simulink library "NeuroMuscularLibrary2"  (R2019b)
settings: Solver=ode45  StartTime=0.0  StopTime=10.0  RelTol=1e-3  EnableMultiTasking=on
values from neighbouring files (symbols this model uses):
  c = 0.05    [BodyMechParams.m]
  c_jointstop = 0.3 / (pi/180)    (= 17.1887338539)    [BodyMechParams.m]
  deltaLegAngleThr = 8*pi/180    (= 0.13962634016)    [CMGParams.m]
  DeltaThRef = 2e-3    (= 0.002)    [BodyMechParams.m]
  eref = 0.04    [BodyMechParams.m]
  FmaxGLU = 1500    [BodyMechParams.m]
  footBallToAnkleDist = 0.16    [BodyMechParams.m]
  footBallToCenterDist = footLength/2    (= 0.1)    [BodyMechParams.m]
  footBallToHeelDist = footLength    (= 0.2)    [BodyMechParams.m]
  footCenterToCGDist = 0.14 - footBallToCenterDist    (= 0.04)    [BodyMechParams.m]
  footInertia = 0.005    [BodyMechParams.m]
  footLength = 0.2    [BodyMechParams.m]
  footMass = 1.25    [BodyMechParams.m]
  FT_GLU = 47.6    [BodyMechParams.m]
  g = 9.80665    [BodyMechParams.m]
  groundTheta = [atan(diff(groundZ)./diff(groundX)), 0]    [generateGround.m]
  groundZ = groundZ * stepSize/(largestStep+eps)    [generateGround.m]
  hatHipToCenterDistLen = hatLength/2    (= 0.4)    [BodyMechParams.m]
  hatInertia = 3    [BodyMechParams.m]
  hatLeftHipToCenterDistWidth = .15    (= 0.15)    [BodyMechParams.m]
  hatLength = 0.8    [BodyMechParams.m]
  hatMass = 53.5    [BodyMechParams.m]
  hatThickness = 0.2    [BodyMechParams.m]
  hatWidth = 0.4    [BodyMechParams.m]
  K = 5    [BodyMechParams.m]
  k_gn = k_gn/2    (= 39226.6)    [BodyMechParams.m]
  k_gt = k_gt/2    (= 39226.6)    [BodyMechParams.m]
  k_pressure = hatMass * g / DeltaThRef    (= 262327.8875)    [BodyMechParams.m]
  legAngleSpeedMax = 10    [CMGParams.m]
  loptGAS = 0.05    [BodyMechParams.m]
  loptGLU = 0.11    [BodyMechParams.m]
  loptHAB = 0.09    [BodyMechParams.m]
  loptHAD = 0.10    (= 0.1)    [BodyMechParams.m]
  loptHAM = 0.10    (= 0.1)    [BodyMechParams.m]
  loptHFL = 0.11    [BodyMechParams.m]
  loptSOL = 0.04    [BodyMechParams.m]
  loptTA = 0.06    [BodyMechParams.m]
  loptVAS = 0.08    [BodyMechParams.m]
  lslackGAS = 0.40    (= 0.4)    [BodyMechParams.m]
  lslackGLU = 0.13    [BodyMechParams.m]
  lslackHAB = 0.07    [BodyMechParams.m]
  lslackHAD = 0.18    [BodyMechParams.m]
  lslackHAM = 0.31    [BodyMechParams.m]
  lslackHFL = 0.10    (= 0.1)    [BodyMechParams.m]
  lslackSOL = 0.26    [BodyMechParams.m]
  lslackTA = 0.24    [BodyMechParams.m]
  lslackVAS = 0.23    [BodyMechParams.m]
  mu_slide = 0.8    [BodyMechParams.m]
  mu_stick = 0.9    [BodyMechParams.m]
  N = 1.5    [BodyMechParams.m]    (also in cmaes.m = size(x,1); mergeCompareEnergyCosts.m = {S.name})
  phiKneeUpLimit = 5*pi/180    (= 0.0872664625997)    [BodyMechParams.m]
  phimaxGASa = 20*pi/180    (= 0.349065850399)    [BodyMechParams.m]
  phimaxGASk = 40*pi/180    (= 0.698131700798)    [BodyMechParams.m]
  phimaxHAMk = 0*pi/180    (= 0)    [BodyMechParams.m]
  phimaxSOL = 20*pi/180    (= 0.349065850399)    [BodyMechParams.m]
  phimaxTA = -10*pi/180    (= -0.174532925199)    [BodyMechParams.m]
  phimaxVAS = 15*pi/180    (= 0.261799387799)    [BodyMechParams.m]
  phirefGASa = -10*pi/180    (= -0.174532925199)    [BodyMechParams.m]
  phirefGASk = 15*pi/180    (= 0.261799387799)    [BodyMechParams.m]
  phirefGLU = -30*pi/180    (= -0.523598775598)    [BodyMechParams.m]
  phirefHAB = 10*pi/180    (= 0.174532925199)    [BodyMechParams.m]
  phirefHAD = 15*pi/180    (= 0.261799387799)    [BodyMechParams.m]
  phirefHAMh = -25*pi/180    (= -0.436332312999)    [BodyMechParams.m]
  phirefHAMk = 0*pi/180    (= 0)    [BodyMechParams.m]
  phirefHFL = 0*pi/180    (= 0)    [BodyMechParams.m]
  phirefSOL = -10*pi/180    (= -0.174532925199)    [BodyMechParams.m]
  phirefTA = 20*pi/180    (= 0.349065850399)    [BodyMechParams.m]
  phirefVAS = 55*pi/180    (= 0.959931088597)    [BodyMechParams.m]
  rGASa = 0.05    [BodyMechParams.m]
  rGASk = 0.05    [BodyMechParams.m]
  rGLU = 0.10    (= 0.1)    [BodyMechParams.m]
  rHAB = 0.06    [BodyMechParams.m]
  rHAD = 0.03    [BodyMechParams.m]
  rHAMh = 0.08    [BodyMechParams.m]
  rHAMk = 0.05    [BodyMechParams.m]
  rHFL = 0.10    (= 0.1)    [BodyMechParams.m]
  rhoGASa = 0.7    [BodyMechParams.m]
  rhoGASk = 0.7    [BodyMechParams.m]
  rhoGLU = 0.5    [BodyMechParams.m]
  rhoHAB = 0.7    [BodyMechParams.m]
  rhoHAD = 1    [BodyMechParams.m]
  rhoHAMh = 0.7    [BodyMechParams.m]
  rhoHAMk = 0.7    [BodyMechParams.m]
  rhoHFL = 0.5    [BodyMechParams.m]
  rhoSOL = 0.5    [BodyMechParams.m]
  rhoTA = 0.7    [BodyMechParams.m]
  rhoVAS = 0.7    [BodyMechParams.m]
  RkneeExtendGain = 25000    [CMGParams.m]
  RkneeStopGain = 12000    [CMGParams.m]
  RlegAngleFilter = 100    [CMGParams.m]
  rSOL = 0.05    [BodyMechParams.m]
  rTA = 0.04    [BodyMechParams.m]
  rVAS = 0.06    [BodyMechParams.m]
  s = x(1:N-1,:).^2 + x(2:N,:).^2    [cmaes.m]
  shankAnkleToCenterDist = shankLength/2    (= 0.25)    [BodyMechParams.m]
  shankAnkleToKneeDist = shankLength    (= 0.5)    [BodyMechParams.m]
  shankCenterToCGDist = 0.3 - shankAnkleToCenterDist    (= 0.05)    [BodyMechParams.m]
  shankInertia = 0.05    [BodyMechParams.m]
  shankLength = 0.5    [BodyMechParams.m]
  shankMass = 3.5    [BodyMechParams.m]
  tau = 0.01    [BodyMechParams.m]
  thighCenterToCGDist = 0.3 - thighKneeToCenterDist    (= 0.05)    [BodyMechParams.m]
  thighInertia = 0.15    [BodyMechParams.m]
  thighKneeToCenterDist = thighLength/2    (= 0.25)    [BodyMechParams.m]
  thighKneeToHipDist = thighLength    (= 0.5)    [BodyMechParams.m]
  thighLength = 0.5    [BodyMechParams.m]
  thighMass = 8.5    [BodyMechParams.m]
  v_gn_max = v_gz_max    (= 0.03)    [BodyMechParams.m]
  v_gt_max = v_gz_max    (= 0.03)    [BodyMechParams.m]
  v_max_pressure = 0.5    [BodyMechParams.m]
  vLimit = 0.01    [BodyMechParams.m]
  w = 0.56    [BodyMechParams.m]    (also in MuscleEnergyTest.m = 1.039; cmaes.m = ones(size(x,1)))
  w_max_jointstop = 1 * pi/180    (= 0.0174532925199)    [BodyMechParams.m]
  X = contains(N,'compareEnergyCost') .* ~contains(N,'total') .* ~contains(N,'Total')    [mergeCompareEnergyCosts.m]
undefined symbols (not defined in the file or in its folder): abdHATRef, ankleBackDriveGain, ankleCJointstop, ankleDgain, ankleFilterPID, ankleFilterSEA, ankleGearEff, ankleGearRatio, ankleIgain, ankleInitialAngle, ankleInputMass, ankleIntCoulomb, ankleIntDamping, ankleIntStatic, ankleParallelSpringDamping, ankleParallelSpringOffset, ankleParallelSpringStiffness, anklePgain, anklePlantarLimit, ankleSEADamping, ankleSEAStiffness, ankleTendonMass, ankleWMaxJointstop, dryFrictionDamping, dryFrictionStiffness, dryFrictionVelThresh, footMassp, FourBarL1, FourBarL3, GainCHAB, GainCHAD, GainGAS, GainGLU, GainHAM, GainKneeOverExt, GainSOL, GainSOLTA, GainTA, GainVAS, hipDGain, hipDGainAbd, hipPGain, hipPGainAbd, Kglu, kneeAngleOffset, kneeBackDriveGain, kneeCJointstop, kneeDgain, kneeExtCoulomb, kneeExtDamping, kneeExtendGain, kneeExtStatic, kneeFilterPID, kneeFilterSEA, kneeFlexGain, kneeGearEff, kneeGearRatio, kneeHoldGain1, kneeHoldGain2, kneeIgain ... (+62)
libraries: sm_lib x105, nesl_utility x55, simulink x22, dspswit3 x15, $bdroot x12, simulink_extras x2
(part 3 of 6)

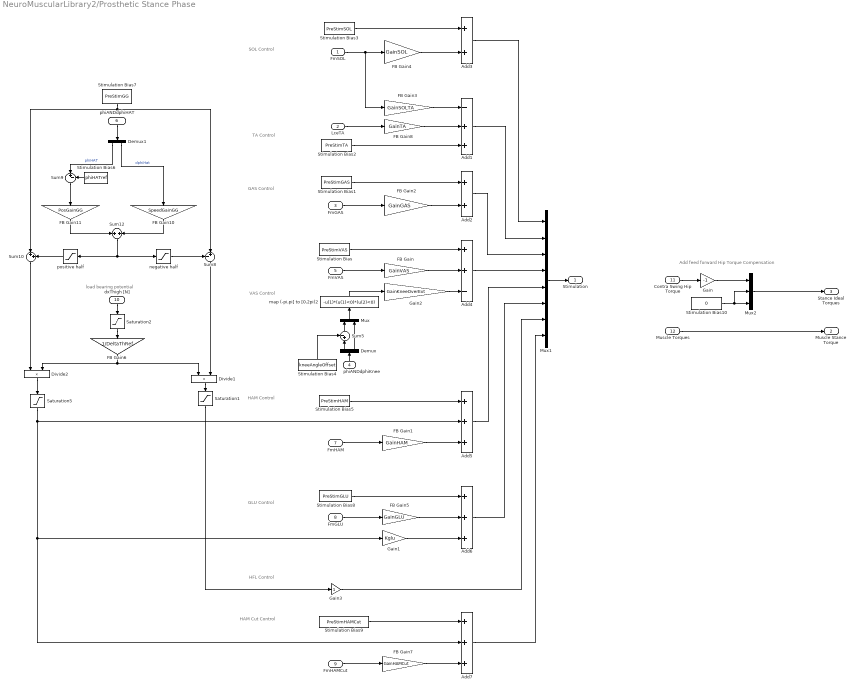
== system NeuroMuscularLibrary2/Prosthetic Stance Phase ==
  note: Add feed forward Hip Torque Compensation
  note: load bearing potential
  note: HFL Control
  note: GLU Control
  note: VAS Control
  note: HAM Control
  note: GAS Control
  note: TA Control
  note: SOL Control
  note: HAM Cut Control
  FmSOL : Inport
  LceTA : Inport  Port=2
  FmGAS : Inport  Port=3
  phiANDdphiKnee : Inport  Port=4
  FmVAS : Inport  Port=5
  phiANDdphiHAT : Inport  Port=6
  FmHAM : Inport  Port=7
  FmGLU : Inport  Port=8
  FmHAMCut : Inport  Port=9
  dxThigh [N] : Inport  Port=10
  Contra Swing Hip Torque : Inport  Port=11
  Muscle Torques : Inport  Port=12
  Add1 : Sum  Inputs=-++
  Add2 : Sum
  Add3 : Sum
  Add4 : Sum  Inputs=++-
  Add5 : Sum  Inputs=+++
  Add6 : Sum  Inputs=+++
  Add7 : Sum  Inputs=+++
  Demux : Demux  Outputs=2
  Demux1 : Demux  Outputs=2
  Divide1 : Product
  Divide2 : Product
  FB Gain : Gain  Gain=GainVAS  SaturateOnIntegerOverflow=on  OutDataTypeStr=Inherit: Same as input  ParamDataTypeStr=Inherit: Same as input
  FB Gain1 : Gain  Gain=GainHAM  SaturateOnIntegerOverflow=on  OutDataTypeStr=Inherit: Same as input  ParamDataTypeStr=Inherit: Same as input
  FB Gain10 : Gain  Gain=SpeedGainGG  SaturateOnIntegerOverflow=on  OutDataTypeStr=Inherit: Same as input  ParamDataTypeStr=Inherit: Same as input
  FB Gain11 : Gain  Gain=PosGainGG  SaturateOnIntegerOverflow=on  OutDataTypeStr=Inherit: Same as input  ParamDataTypeStr=Inherit: Same as input
  FB Gain2 : Gain  Gain=GainGAS  SaturateOnIntegerOverflow=on  OutDataTypeStr=Inherit: Same as input  ParamDataTypeStr=Inherit: Same as input
  FB Gain3 : Gain  Gain=GainSOLTA  SaturateOnIntegerOverflow=on  OutDataTypeStr=Inherit: Same as input  ParamDataTypeStr=Inherit: Same as input
  FB Gain4 : Gain  Gain=GainSOL  SaturateOnIntegerOverflow=on  OutDataTypeStr=Inherit: Same as input  ParamDataTypeStr=Inherit: Same as input
  FB Gain5 : Gain  Gain=GainGLU  SaturateOnIntegerOverflow=on  OutDataTypeStr=Inherit: Same as input  ParamDataTypeStr=Inherit: Same as input
  FB Gain6 : Gain  Gain=1/DeltaThRef  SaturateOnIntegerOverflow=on  OutDataTypeStr=Inherit: Same as input  ParamDataTypeStr=Inherit: Same as input
  FB Gain7 : Gain  Gain=GainHAMCut  SaturateOnIntegerOverflow=on  OutDataTypeStr=Inherit: Same as input  ParamDataTypeStr=Inherit: Same as input
  FB Gain8 : Gain  Gain=GainTA  SaturateOnIntegerOverflow=on  OutDataTypeStr=Inherit: Same as input  ParamDataTypeStr=Inherit: Same as input
  Gain : Gain  Gain=-1
  Gain1 : Gain  Gain=Kglu
  Gain2 : Gain  Gain=GainKneeOverExt
  Gain3 : Gain
  Mux : Mux  Inputs=2
  Mux1 : Mux  Inputs=8
  Mux2 : Mux  Inputs=3
  Saturation1 : Saturate  UpperLimit=1  LowerLimit=0  ZeroCross=off
  Saturation2 : Saturate  UpperLimit=inf  LowerLimit=0  ZeroCross=off
  Saturation5 : Saturate  UpperLimit=1  LowerLimit=0  ZeroCross=off
  Stimulation Bias : Constant  Value=PreStimVAS
  Stimulation Bias1 : Constant  Value=PreStimGAS
  Stimulation Bias10 : Constant  Value=0
  Stimulation Bias2 : Constant  Value=PreStimTA
  Stimulation Bias3 : Constant  Value=PreStimSOL
  Stimulation Bias4 : Constant  Value=kneeAngleOffset
  Stimulation Bias5 : Constant  Value=PreStimHAM
  Stimulation Bias6 : Constant  Value=phiHATref
  Stimulation Bias7 : Constant  Value=PreStimGG
  Stimulation Bias8 : Constant  Value=PreStimGLU
  Stimulation Bias9 : Constant  Value=PreStimHAMCut
  Sum10 : Sum  Inputs=|++  SaturateOnIntegerOverflow=on  InputSameDT=on  OutDataTypeStr=Inherit: Same as first input
  Sum12 : Sum  SaturateOnIntegerOverflow=on  InputSameDT=on  OutDataTypeStr=Inherit: Same as first input
  Sum5 : Sum  Inputs=-+|  SaturateOnIntegerOverflow=on  InputSameDT=on  OutDataTypeStr=Inherit: Same as first input
  Sum8 : Sum  Inputs=-+|  SaturateOnIntegerOverflow=on  InputSameDT=on  OutDataTypeStr=Inherit: Same as first input
  Sum9 : Sum  Inputs=|+-  SaturateOnIntegerOverflow=on  InputSameDT=on  OutDataTypeStr=Inherit: Same as first input
  map (-pi,pi] to [0,2pi)2 : Fcn  Expr=-u(1)*(u(1)<0)*(u(2)<0)
  negative half : Saturate  UpperLimit=0  LowerLimit=-inf  ZeroCross=off
  positive half : Saturate  UpperLimit=inf  LowerLimit=0  ZeroCross=off
  Stimulation : Outport
  Muscle Stance Torque : Outport  Port=2
  Stance Ideal Torques : Outport  Port=3
  wires:
  Muscle Torques/1 -> Muscle Stance Torque/1
  Mux2/1 -> Stance Ideal Torques/1
  Stimulation Bias10/1 -> Mux2/2, Mux2/3
  Contra Swing Hip Torque/1 -> Gain/1
  Gain/1 -> Mux2/1
  Add4/1 -> Mux1/4
  Mux1/1 -> Stimulation/1
  Gain1/1 -> Add6/3
  FB Gain5/1 -> Add6/2
  Stimulation Bias8/1 -> Add6/1
  Add6/1 -> Mux1/6
  Add5/1 -> Mux1/5
  FB Gain1/1 -> Add5/3
  Stimulation Bias5/1 -> Add5/1
  Stimulation Bias/1 -> Add4/1
  Stimulation Bias1/1 -> Add2/1
  Add2/1 -> Mux1/3
  Stimulation Bias2/1 -> Add1/3
  Stimulation Bias3/1 -> Add3/1
  FmGLU/1 -> FB Gain5/1
  FmHAM/1 -> FB Gain1/1
  map (-pi,pi] to [0,2pi)2/1 -> Gain2/1
  Sum8/1 -> Divide1/2
  Sum10/1 -> Divide2/1
  Sum9/1 -> FB Gain11/1
  FB Gain6/1 -> Divide1/1, Divide2/2
  Divide2/1 -> Saturation5/1
  Divide1/1 -> Saturation1/1
  Saturation1/1 -> Gain3/1
  dxThigh [N]/1 -> Saturation2/1
  Saturation2/1 -> FB Gain6/1
  Gain3/1 -> Mux1/7
  Gain2/1 -> Add4/3
  negative half/1 -> Sum8/1
  Sum12/1 -> negative half/1, positive half/1
  positive half/1 -> Sum10/2
  Demux1/2 -> FB Gain10/1  "dphiHat"
  Demux1/1 -> Sum9/1  "phiHAT"
  phiANDdphiHAT/1 -> Demux1/1
  FB Gain10/1 -> Sum12/2
  FB Gain11/1 -> Sum12/1
  Stimulation Bias7/1 -> Sum8/2, Sum10/1
  Stimulation Bias6/1 -> Sum9/2
  Stimulation Bias4/1 -> Sum5/1
  Demux/2 -> Mux/2
  Demux/1 -> Sum5/2
  phiANDdphiKnee/1 -> Demux/1
  Sum5/1 -> Mux/1
  Mux/1 -> map (-pi,pi] to [0,2pi)2/1
  FmVAS/1 -> FB Gain/1
  FB Gain/1 -> Add4/2
  FB Gain2/1 -> Add2/2
  FmGAS/1 -> FB Gain2/1
  LceTA/1 -> FB Gain8/1
  FB Gain8/1 -> Add1/2
  Add1/1 -> Mux1/2
  FB Gain3/1 -> Add1/1
  FmSOL/1 -> FB Gain3/1, FB Gain4/1
  FB Gain4/1 -> Add3/2
  Add3/1 -> Mux1/1
  Add7/1 -> Mux1/8
  FB Gain7/1 -> Add7/3
  Stimulation Bias9/1 -> Add7/1
  FmHAMCut/1 -> FB Gain7/1
  Saturation5/1 -> Add5/2, Add7/2, Gain1/1

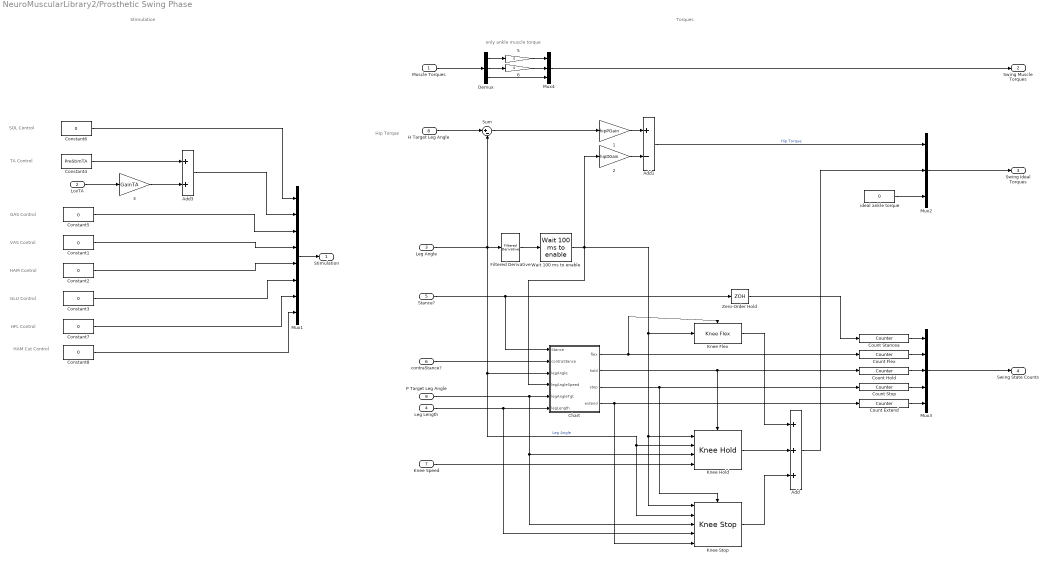
== system NeuroMuscularLibrary2/Prosthetic Swing Phase ==
  note: Hip Torque
  note: only ankle muscle torque
  note: HAM Cut
      | Control
  note: Torques
  note: HFL Control
  note: GLU Control
  note: HAM Control
  note: VAS Control
  note: TA Control
  note: GAS Control
  note: SOL Control
  note: Stimulation
  Muscle Torques : Inport
  LceTA : Inport  Port=2
  Leg Angle : Inport  Port=3
  Leg Length : Inport  Port=4
  Stance? : Inport  Port=5
  contraStance? : Inport  Port=6
  Knee Speed : Inport  Port=7
  H Target Leg Angle : Inport  Port=8
  P Target Leg Angle : Inport  Port=9
  " 1" : Gain  Gain=hipPGain
  " 2" : Gain  Gain=hipDGain
  " 3" : Gain  Gain=GainTA
  " 5" : Gain  Gain=0
  " 6" : Gain  Gain=0
  Add : Sum  Inputs=+++
  Add1 : Sum  Inputs=+-
  Add3 : Sum
  Chart : Stateflow chart  TreatAsAtomicUnit=on
  Constant{1..3,5..8} (7 alike) : Constant  Value=0
  Constant4 : Constant  Value=PreStimTA
  Count Extend : dspswit3/Counter  Direction=Up  CountEvent=Rising edge  CounterSize=16 bits  MaxCount=255  InitialCount=0  Output=Count  HitValue=32  ResetInput=off  SamplesPerFrame=1  Ts=1  CntDtype=double  HitDtype=Logical
  Count Flex : dspswit3/Counter  Direction=Up  CountEvent=Rising edge  CounterSize=16 bits  MaxCount=255  InitialCount=0  Output=Count  HitValue=32  ResetInput=off  SamplesPerFrame=1  Ts=1  CntDtype=double  HitDtype=Logical
  Count Hold : dspswit3/Counter  Direction=Up  CountEvent=Rising edge  CounterSize=16 bits  MaxCount=255  InitialCount=0  Output=Count  HitValue=32  ResetInput=off  SamplesPerFrame=1  Ts=1  CntDtype=double  HitDtype=Logical
  Count Stancea : dspswit3/Counter  Direction=Up  CountEvent=Rising edge  CounterSize=16 bits  MaxCount=255  InitialCount=0  Output=Count  HitValue=32  ResetInput=off  SamplesPerFrame=1  Ts=1  CntDtype=double  HitDtype=Logical
  Count Stop : dspswit3/Counter  Direction=Up  CountEvent=Rising edge  CounterSize=16 bits  MaxCount=255  InitialCount=0  Output=Count  HitValue=32  ResetInput=off  SamplesPerFrame=1  Ts=1  CntDtype=double  HitDtype=Logical
  Demux : Demux  Outputs=3
  Filtered Derivative : $bdroot/Swing Phase/Filtered Derivative  SystemSampleTime=-1  Latency=0  AutoFrameSizeCalculation=off
  Knee Flex : $bdroot/Swing Phase/Knee Flex  SystemSampleTime=-1  Latency=0  AutoFrameSizeCalculation=off
  Knee Hold : $bdroot/Swing Phase/Knee Hold  SystemSampleTime=-1  Latency=0  AutoFrameSizeCalculation=off
  Knee Stop : $bdroot/Swing Phase/Knee Stop  SystemSampleTime=-1  Latency=0  AutoFrameSizeCalculation=off
  Mux1 : Mux  Inputs=8
  Mux2 : Mux  Inputs=3
  Mux3 : Mux  Inputs=5
  Mux4 : Mux  Inputs=3
  Sum : Sum  Inputs=|+-
  Wait 100 ms to enable : $bdroot/Swing Phase/Wait 100 ms to enable  SystemSampleTime=-1  Latency=0  AutoFrameSizeCalculation=off
  Zero-Order Hold : ZeroOrderHold  SampleTime=.01
  ideal ankle torque : Constant  Value=0
  Stimulation : Outport
  Swing Muscle Torques : Outport  Port=2
  Swing Ideal Torques : Outport  Port=3
  Swing State Counts : Outport  Port=4
  wires:
  P Target Leg Angle/1 -> Chart/5(legAngleTgt), Knee Hold/3, Knee Stop/3
  Mux2/1 -> Swing Ideal Torques/1
  ideal ankle torque/1 -> Mux2/3
  Zero-Order Hold/1 -> Count Stancea/1
  Count Stancea/1 -> Mux3/1
  Mux3/1 -> Swing State Counts/1
  Count Flex/1 -> Mux3/2
  Count Hold/1 -> Mux3/3
  Count Stop/1 -> Mux3/4
  Count Extend/1 -> Mux3/5
  Add1/1 -> Mux2/1  "Hip Torque"
  Leg Length/1 -> Knee Stop/4, Chart/6(legLength)
  contraStance?/1 -> Chart/2(contraStance)
  Stance?/1 -> Chart/1(Stance), Zero-Order Hold/1
  Chart/4(extend) -> Knee Stop/5, Count Extend/1
  Chart/3(stop) -> Knee Stop/Enable, Count Stop/1
  Chart/2(hold) -> Knee Hold/Enable, Count Hold/1
  Chart/1(flex) -> Count Flex/1, Knee Flex/Enable
  Add/1 -> Mux2/2
  Knee Stop/1 -> Add/3
  Knee Flex/1 -> Add/1
  Knee Hold/1 -> Add/2
  Knee Speed/1 -> Knee Hold/4
  Leg Angle/1 -> Sum/2, Knee Hold/2, Knee Stop/2, Chart/3(legAngle), Filtered Derivative/1  "Leg Angle"
  Sum/1 -> " 1"/1
  " 1"/1 -> Add1/1
  " 2"/1 -> Add1/2
  H Target Leg Angle/1 -> Sum/1
  Filtered Derivative/1 -> Wait 100 ms to enable/1
  Wait 100 ms to enable/1 -> " 2"/1, Knee Flex/1, Knee Stop/1, Knee Hold/1, Chart/4(legAngleSpeed)
  Demux/3 -> Mux4/3
  " 6"/1 -> Mux4/2
  " 5"/1 -> Mux4/1
  Demux/2 -> " 6"/1
  Demux/1 -> " 5"/1
  Muscle Torques/1 -> Demux/1
  Mux4/1 -> Swing Muscle Torques/1
  Constant8/1 -> Mux1/8
  Mux1/1 -> Stimulation/1
  Constant7/1 -> Mux1/7
  Constant3/1 -> Mux1/6
  Constant2/1 -> Mux1/5
  Constant1/1 -> Mux1/4
  Constant5/1 -> Mux1/3
  Constant6/1 -> Mux1/1
  Add3/1 -> Mux1/2
  LceTA/1 -> " 3"/1
  " 3"/1 -> Add3/2
  Constant4/1 -> Add3/1

== system NeuroMuscularLibrary2/SOL Link ==
  note: Soleus Attachment
  Ankle Angle [rad] : Inport
  Constant : Constant  Value=lslackSOL+loptSOL
  Constant2 : Constant  Value=phirefSOL
  Constant3 : Constant  Value=phimaxSOL
  Demux : Demux  Outputs=2
  Gain2 : Gain  Gain=rSOL
  Gain4 : Gain  Gain=rhoSOL
  Mux : Mux  Inputs=2
  Sum2 : Sum  Inputs=|+-
  Sum3 : Sum  Inputs=-+|
  Sum4 : Sum  Inputs=+-
  Sum5 : Sum  Inputs=|++
  length change term : Trigonometry
  offset correction term : Trigonometry
  variable lever term : Trigonometry  Operator=cos
  lmtc [m] : Outport
  lever [m] : Outport  Port=2
  wires:
  Ankle Angle [rad]/1 -> Sum3/2
  Sum3/1 -> variable lever term/1, length change term/1
  Constant3/1 -> Sum3/1, Sum2/2
  Sum2/1 -> offset correction term/1
  Constant2/1 -> Sum2/1
  length change term/1 -> Sum4/2
  offset correction term/1 -> Sum4/1
  Sum4/1 -> Mux/1
  Constant/1 -> Sum5/1
  Sum5/1 -> lmtc [m]/1
  Gain4/1 -> Sum5/2
  variable lever term/1 -> Mux/2
  Mux/1 -> Gain2/1
  Gain2/1 -> Demux/1
  Demux/1 -> Gain4/1
  Demux/2 -> lever [m]/1

== system NeuroMuscularLibrary2/Sensor Sheet ==
  note: Inner Segment Pressure Sheet
  Gain3 : Gain  Gain=k_pressure
  Gain4 : Gain  Gain=1/v_max_pressure
  Mux1 : Mux  Inputs=2
  PS-Simulink Converter : nesl_utility/PS-Simulink Converter  PhysicalDomain=network_engine_domain  SubClassName=ps_output  LeftPortType=input  RightPortType=output  PseudoPeriodic=off  Frequencies=[]  Unit=1  AffineConversion=off
  PS-Simulink Converter1 : nesl_utility/PS-Simulink Converter  PhysicalDomain=network_engine_domain  SubClassName=ps_output  LeftPortType=input  RightPortType=output  PseudoPeriodic=off  Frequencies=[]  Unit=1  AffineConversion=off
  Pressure Sheet Reaction Force : Fcn  Expr=-u(1) * (1+sgn(u(1))*u(2))
  Prismatic Joint : sm_lib/Joints/Prismatic Joint  JointMode=Normal  SenseConstraintForce=off  SenseConstraintForceX=off  SenseConstraintForceY=off  SenseConstraintForceZ=off  SenseConstraintTorque=off  SenseConstraintTorqueX=off  SenseConstraintTorqueY=off  SenseConstraintTorqueZ=off  SenseTotalForce=off  SenseTotalForceX=off  SenseTotalForceY=off  SenseTotalForceZ=off  SenseTotalTorque=off  SenseTotalTorqueX=off  SenseTotalTorqueY=off  SenseTotalTorqueZ=off  CompositeWrenchDir=FollowerOnBase  CompositeWrenchFrame=BaseFrame  EquilibriumPosition=0  EquilibriumPositionUnits=m  SpringStiffness=0  SpringStiffnessUnits=N/m  DampingCoefficient=0  DampingCoefficientUnits=N/(m/s)  TorqueActuationMode=InputTorque  MotionActuationMode=ComputedMotion  SensePosition=on  SenseVelocity=on  SenseAcceleration=off  SenseTorqueForce=off  SenseLowerLimitTorqueForce=off  SenseUpperLimitTorqueForce=off  LowerLimitSpecify=off  LowerLimitBound=-1  LowerLimitBoundUnits=m  LowerLimitStiffness=1e6  LowerLimitStiffnessUnits=N/m  LowerLimitDamping=1e3  LowerLimitDampingUnits=N/(m/s)  LowerLimitTransitionRegionWidth=1e-4  LowerLimitTransitionRegionWidthUnits=m  UpperLimitSpecify=off  UpperLimitBound=1  UpperLimitBoundUnits=m  UpperLimitStiffness=1e6  UpperLimitStiffnessUnits=N/m  UpperLimitDamping=1e3  UpperLimitDampingUnits=N/(m/s)  UpperLimitTransitionRegionWidth=1e-4  UpperLimitTransitionRegionWidthUnits=m  PositionTargetSpecify=on  PositionTargetPriority=High  PositionTargetValue=0  PositionTargetValueUnits=m  VelocityTargetSpecify=on  VelocityTargetPriority=High  VelocityTargetValue=0  VelocityTargetValueUnits=m/s
  Simulink-PS Converter : nesl_utility/Simulink-PS Converter  PhysicalDomain=network_engine_domain  SubClassName=ps_input  LeftPortType=input  RightPortType=output  PseudoPeriodic=off  Frequencies=[]  NoiseDistribution=none  NoiseParameters=[]  Unit=1  AffineConversion=off  FilteringAndDerivatives=zero  SimscapeFilterOrder=1  InputFilterTimeConstant=0.001  UdotUserProvided=1
  Y-up TO Z-up : sm_lib/Frames and Transforms/Rigid Transform  TranslationMethod=None  TranslationStandardOffset=0  TranslationLengthUnit=m  TranslationStandardAxis=+Z  TranslationCartesianOffset=[0 0 0]  TranslationROffset=0  TranslationROffsetUnits=m  TranslationZOffset=0  TranslationZOffsetUnits=m  TranslationThetaOffset=0  TranslationThetaOffsetUnits=deg  RotationMethod=AlignedAxes  RotationAngleUnits=deg  RotationStandardAxis=+Z  RotationAngle=0  RotationArbitraryAxis=[0 0 1]  FollAlignAxisA=+X  BaseAlignAxisA=+X  FollAlignAxisB=+Z  BaseAlignAxisB=+Y  RotationSequenceAxes=FollowerAxes  RotationSequence=XYX  RotationSequenceAngles=[0 0 0]  RotationSequenceAnglesUnits=deg  RotationMatrix=[1 0 0; 0 1 0; 0 0 1]
  Z-up TO Y-up : sm_lib/Frames and Transforms/Rigid Transform  TranslationMethod=None  TranslationStandardOffset=0  TranslationLengthUnit=m  TranslationStandardAxis=+Z  TranslationCartesianOffset=[0 0 0]  TranslationROffset=0  TranslationROffsetUnits=m  TranslationZOffset=0  TranslationZOffsetUnits=m  TranslationThetaOffset=0  TranslationThetaOffsetUnits=deg  RotationMethod=AlignedAxes  RotationAngleUnits=deg  RotationStandardAxis=+Z  RotationAngle=0  RotationArbitraryAxis=[0 0 1]  FollAlignAxisA=+X  BaseAlignAxisA=+X  FollAlignAxisB=+Y  BaseAlignAxisB=+Z  RotationSequenceAxes=FollowerAxes  RotationSequence=XYX  RotationSequenceAngles=[0 0 0]  RotationSequenceAnglesUnits=deg  RotationMatrix=[1 0 0; 0 1 0; 0 0 1]
  Thigh : PMIOPort  Side=Left
  Hip Joint : PMIOPort  Port=2  Side=Right
  dx : Outport
  wires:
  PS-Simulink Converter/1 -> Gain3/1, dx/1  "position"
  PS-Simulink Converter1/1 -> Gain4/1  "velocity"
  Mux1/1 -> Pressure Sheet Reaction Force/1
  Gain3/1 -> Mux1/1
  Gain4/1 -> Mux1/2
  Pressure Sheet Reaction Force/1 -> Simulink-PS Converter/1
  connections:
  Prismatic Joint/LConn1 -- Y-up TO Z-up/RConn1
  Prismatic Joint/RConn1 -- Z-up TO Y-up/LConn1
  Prismatic Joint/LConn2 -- Simulink-PS Converter/RConn1
  Prismatic Joint/RConn2 -- PS-Simulink Converter/LConn1
  Prismatic Joint/RConn3 -- PS-Simulink Converter1/LConn1
  Y-up TO Z-up/LConn1 -- Thigh/RConn1
  Hip Joint/RConn1 -- Z-up TO Y-up/RConn1

== system NeuroMuscularLibrary2/Shank ==
  Ankle to Center : sm_lib/Frames and Transforms/Rigid Transform  TranslationMethod=Cartesian  TranslationStandardOffset=0  TranslationLengthUnit=m  TranslationStandardAxis=+Z  TranslationCartesianOffset=[0 shankAnkleToCenterDist 0]  TranslationROffset=0  TranslationROffsetUnits=m  TranslationZOffset=0  TranslationZOffsetUnits=m  TranslationThetaOffset=0  TranslationThetaOffsetUnits=deg  RotationMethod=AlignedAxes  RotationAngleUnits=deg  RotationStandardAxis=+Z  RotationAngle=0  RotationArbitraryAxis=[0 0 1]  FollAlignAxisA=+Z  BaseAlignAxisA=+Y  FollAlignAxisB=+X  BaseAlignAxisB=+X  RotationSequenceAxes=FollowerAxes  RotationSequence=XYX  RotationSequenceAngles=[0 0 0]  RotationSequenceAnglesUnits=deg  RotationMatrix=[1 0 0; 0 1 0; 0 0 1]
  Ankle to Knee : sm_lib/Frames and Transforms/Rigid Transform  TranslationMethod=Cartesian  TranslationStandardOffset=0  TranslationLengthUnit=m  TranslationStandardAxis=+Z  TranslationCartesianOffset=[0 shankAnkleToKneeDist 0]  TranslationROffset=0  TranslationROffsetUnits=m  TranslationZOffset=0  TranslationZOffsetUnits=m  TranslationThetaOffset=0  TranslationThetaOffsetUnits=deg  RotationMethod=None  RotationAngleUnits=deg  RotationStandardAxis=+Z  RotationAngle=0  RotationArbitraryAxis=[0 0 1]  FollAlignAxisA=+Z  BaseAlignAxisA=+Z  FollAlignAxisB=+X  BaseAlignAxisB=-X  RotationSequenceAxes=FollowerAxes  RotationSequence=XYX  RotationSequenceAngles=[0 0 0]  RotationSequenceAnglesUnits=deg  RotationMatrix=[1 0 0; 0 1 0; 0 0 1]
  Shank Center to CG : sm_lib/Frames and Transforms/Rigid Transform  TranslationMethod=Cartesian  TranslationStandardOffset=0  TranslationLengthUnit=m  TranslationStandardAxis=+Z  TranslationCartesianOffset=[0 0 shankCenterToCGDist]  TranslationROffset=0  TranslationROffsetUnits=m  TranslationZOffset=0  TranslationZOffsetUnits=m  TranslationThetaOffset=0  TranslationThetaOffsetUnits=deg  RotationMethod=None  RotationAngleUnits=deg  RotationStandardAxis=+Z  RotationAngle=0  RotationArbitraryAxis=[0 0 1]  FollAlignAxisA=+X  BaseAlignAxisA=+Y  FollAlignAxisB=+Y  BaseAlignAxisB=+Z  RotationSequenceAxes=FollowerAxes  RotationSequence=XYX  RotationSequenceAngles=[0 0 0]  RotationSequenceAnglesUnits=deg  RotationMatrix=[1 0 0; 0 1 0; 0 0 1]
  Shank Solid : sm_lib/Body Elements/Cylindrical Solid  GraphicAmbientColor=[0.15 0.15 0.15 1.0]  BasedOnType=Density  CenterOfMass=[0 0 shankCenterToCGDist]  CenterOfMassUnits=m  GraphicDiffuseColor=[0.5 0.5 0.5]  CylinderLength=shankLength  CylinderLengthUnits=m  CylinderRadius=.04  CylinderRadiusUnits=m  Density=1000  DensityUnits=kg/(m^3)  DoExposeReferenceFrame=on  GraphicEmissiveColor=[0.0 0.0 0.0 1.0]  ExportEntireGeometry=off  SerializedFrames=<Frames/>  MarkerShape=Sphere  MarkerSize=10  GraphicType=FromGeometry  InertiaType=Custom  Mass=shankMass  MassUnits=kg  MomentsOfInertia=[shankInertia 0 0]  MomentsOfInertiaUnits=kg*m^2  GraphicOpacity=1.0  ProductsOfInertia=[0 0 0]  ProductsOfInertiaUnits=kg*m^2  GraphicShininess=75  GraphicSpecularColor=[0.5 0.5 0.5 1.0]  GraphicVisPropType=SimpleVisualProperties
  Ankle : PMIOPort  Side=Left
  Knee : PMIOPort  Port=2  Side=Right
  CG : PMIOPort  Port=3  Side=Left
  connections:
  Ankle to Knee/LConn1 -- Ankle/RConn1 -- Ankle to Center/LConn1
  Shank Solid/RConn1 -- Ankle to Center/RConn1 -- Shank Center to CG/LConn1
  Ankle to Knee/RConn1 -- Knee/RConn1
  CG/RConn1 -- Shank Center to CG/RConn1

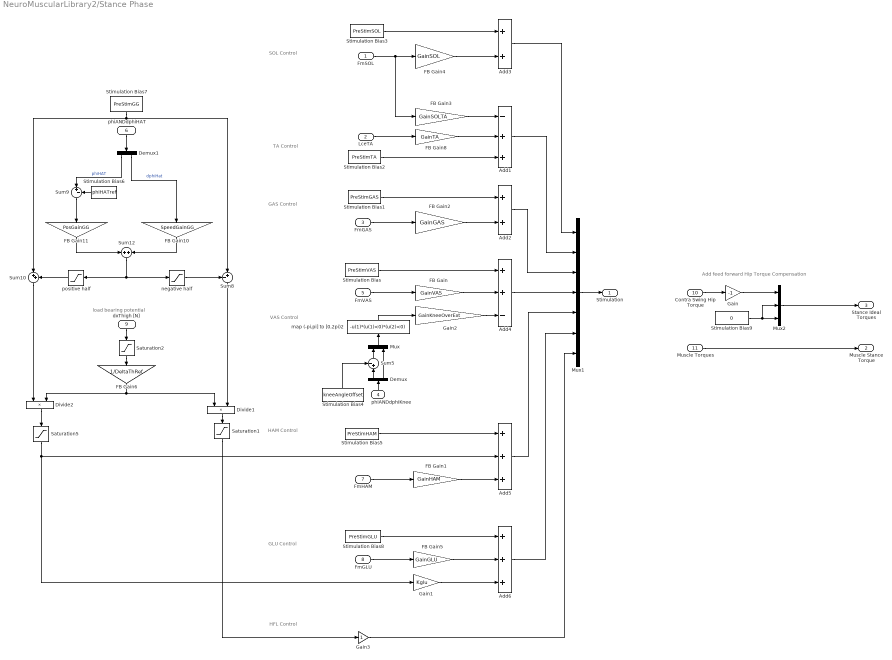
== system NeuroMuscularLibrary2/Stance Phase ==
  note: SOL Control
  note: TA Control
  note: GAS Control
  note: HAM Control
  note: VAS Control
  note: GLU Control
  note: HFL Control
  note: load bearing potential
  note: Add feed forward Hip Torque Compensation
  FmSOL : Inport
  LceTA : Inport  Port=2
  FmGAS : Inport  Port=3
  phiANDdphiKnee : Inport  Port=4
  FmVAS : Inport  Port=5
  phiANDdphiHAT : Inport  Port=6
  FmHAM : Inport  Port=7
  FmGLU : Inport  Port=8
  dxThigh [N] : Inport  Port=9
  Contra Swing Hip Torque : Inport  Port=10
  Muscle Torques : Inport  Port=11
  Add1 : Sum  Inputs=-++
  Add2 : Sum
  Add3 : Sum
  Add4 : Sum  Inputs=++-
  Add5 : Sum  Inputs=+++
  Add6 : Sum  Inputs=+++
  Demux : Demux  Outputs=2
  Demux1 : Demux  Outputs=2
  Divide1 : Product
  Divide2 : Product
  FB Gain : Gain  Gain=GainVAS  SaturateOnIntegerOverflow=on  OutDataTypeStr=Inherit: Same as input  ParamDataTypeStr=Inherit: Same as input
  FB Gain1 : Gain  Gain=GainHAM  SaturateOnIntegerOverflow=on  OutDataTypeStr=Inherit: Same as input  ParamDataTypeStr=Inherit: Same as input
  FB Gain10 : Gain  Gain=SpeedGainGG  SaturateOnIntegerOverflow=on  OutDataTypeStr=Inherit: Same as input  ParamDataTypeStr=Inherit: Same as input
  FB Gain11 : Gain  Gain=PosGainGG  SaturateOnIntegerOverflow=on  OutDataTypeStr=Inherit: Same as input  ParamDataTypeStr=Inherit: Same as input
  FB Gain2 : Gain  Gain=GainGAS  SaturateOnIntegerOverflow=on  OutDataTypeStr=Inherit: Same as input  ParamDataTypeStr=Inherit: Same as input
  FB Gain3 : Gain  Gain=GainSOLTA  SaturateOnIntegerOverflow=on  OutDataTypeStr=Inherit: Same as input  ParamDataTypeStr=Inherit: Same as input
  FB Gain4 : Gain  Gain=GainSOL  SaturateOnIntegerOverflow=on  OutDataTypeStr=Inherit: Same as input  ParamDataTypeStr=Inherit: Same as input
  FB Gain5 : Gain  Gain=GainGLU  SaturateOnIntegerOverflow=on  OutDataTypeStr=Inherit: Same as input  ParamDataTypeStr=Inherit: Same as input
  FB Gain6 : Gain  Gain=1/DeltaThRef  SaturateOnIntegerOverflow=on  OutDataTypeStr=Inherit: Same as input  ParamDataTypeStr=Inherit: Same as input
  FB Gain8 : Gain  Gain=GainTA  SaturateOnIntegerOverflow=on  OutDataTypeStr=Inherit: Same as input  ParamDataTypeStr=Inherit: Same as input
  Gain : Gain  Gain=-1
  Gain1 : Gain  Gain=Kglu
  Gain2 : Gain  Gain=GainKneeOverExt
  Gain3 : Gain
  Mux : Mux  Inputs=2
  Mux1 : Mux  Inputs=7
  Mux2 : Mux  Inputs=3
  Saturation1 : Saturate  UpperLimit=1  LowerLimit=0  ZeroCross=off
  Saturation2 : Saturate  UpperLimit=inf  LowerLimit=0  ZeroCross=off
  Saturation5 : Saturate  UpperLimit=1  LowerLimit=0  ZeroCross=off
  Stimulation Bias : Constant  Value=PreStimVAS
  Stimulation Bias1 : Constant  Value=PreStimGAS
  Stimulation Bias2 : Constant  Value=PreStimTA
  Stimulation Bias3 : Constant  Value=PreStimSOL
  Stimulation Bias4 : Constant  Value=kneeAngleOffset
  Stimulation Bias5 : Constant  Value=PreStimHAM
  Stimulation Bias6 : Constant  Value=phiHATref
  Stimulation Bias7 : Constant  Value=PreStimGG
  Stimulation Bias8 : Constant  Value=PreStimGLU
  Stimulation Bias9 : Constant  Value=0
  Sum10 : Sum  Inputs=|++  SaturateOnIntegerOverflow=on  InputSameDT=on  OutDataTypeStr=Inherit: Same as first input
  Sum12 : Sum  SaturateOnIntegerOverflow=on  InputSameDT=on  OutDataTypeStr=Inherit: Same as first input
  Sum5 : Sum  Inputs=-+|  SaturateOnIntegerOverflow=on  InputSameDT=on  OutDataTypeStr=Inherit: Same as first input
  Sum8 : Sum  Inputs=-+|  SaturateOnIntegerOverflow=on  InputSameDT=on  OutDataTypeStr=Inherit: Same as first input
  Sum9 : Sum  Inputs=|+-  SaturateOnIntegerOverflow=on  InputSameDT=on  OutDataTypeStr=Inherit: Same as first input
  map (-pi,pi] to [0,2pi)2 : Fcn  Expr=-u(1)*(u(1)<0)*(u(2)<0)
  negative half : Saturate  UpperLimit=0  LowerLimit=-inf  ZeroCross=off
  positive half : Saturate  UpperLimit=inf  LowerLimit=0  ZeroCross=off
  Stimulation : Outport
  Muscle Stance Torque : Outport  Port=2
  Stance Ideal Torques : Outport  Port=3
  wires:
  Muscle Torques/1 -> Muscle Stance Torque/1
  Mux2/1 -> Stance Ideal Torques/1
  Stimulation Bias9/1 -> Mux2/2, Mux2/3
  Add3/1 -> Mux1/1
  FB Gain4/1 -> Add3/2
  FmSOL/1 -> FB Gain4/1, FB Gain3/1
  FB Gain3/1 -> Add1/1
  Add1/1 -> Mux1/2
  FB Gain8/1 -> Add1/2
  LceTA/1 -> FB Gain8/1
  FmGAS/1 -> FB Gain2/1
  FB Gain2/1 -> Add2/2
  FB Gain/1 -> Add4/2
  FmVAS/1 -> FB Gain/1
  Mux/1 -> map (-pi,pi] to [0,2pi)2/1
  Sum5/1 -> Mux/1
  phiANDdphiKnee/1 -> Demux/1
  Demux/1 -> Sum5/2
  Demux/2 -> Mux/2
  Stimulation Bias4/1 -> Sum5/1
  Stimulation Bias6/1 -> Sum9/2
  Stimulation Bias7/1 -> Sum10/1, Sum8/2
  FB Gain11/1 -> Sum12/1
  FB Gain10/1 -> Sum12/2
  phiANDdphiHAT/1 -> Demux1/1
  Demux1/1 -> Sum9/1  "phiHAT"
  Demux1/2 -> FB Gain10/1  "dphiHat"
  positive half/1 -> Sum10/2
  Sum12/1 -> positive half/1, negative half/1
  negative half/1 -> Sum8/1
  Gain2/1 -> Add4/3
  Gain3/1 -> Mux1/7
  Saturation2/1 -> FB Gain6/1
  dxThigh [N]/1 -> Saturation2/1
  Saturation1/1 -> Gain3/1
  Divide1/1 -> Saturation1/1
  Divide2/1 -> Saturation5/1
  Saturation5/1 -> Gain1/1, Add5/2
  FB Gain6/1 -> Divide2/2, Divide1/1
  Sum9/1 -> FB Gain11/1
  Sum10/1 -> Divide2/1
  Sum8/1 -> Divide1/2
  map (-pi,pi] to [0,2pi)2/1 -> Gain2/1
  FmHAM/1 -> FB Gain1/1
  FmGLU/1 -> FB Gain5/1
  Stimulation Bias3/1 -> Add3/1
  Stimulation Bias2/1 -> Add1/3
  Add2/1 -> Mux1/3
  Stimulation Bias1/1 -> Add2/1
  Stimulation Bias/1 -> Add4/1
  Stimulation Bias5/1 -> Add5/1
  FB Gain1/1 -> Add5/3
  Add5/1 -> Mux1/5
  Add6/1 -> Mux1/6
  Stimulation Bias8/1 -> Add6/1
  FB Gain5/1 -> Add6/2
  Gain1/1 -> Add6/3
  Mux1/1 -> Stimulation/1
  Add4/1 -> Mux1/4
  Contra Swing Hip Torque/1 -> Gain/1
  Gain/1 -> Mux2/1

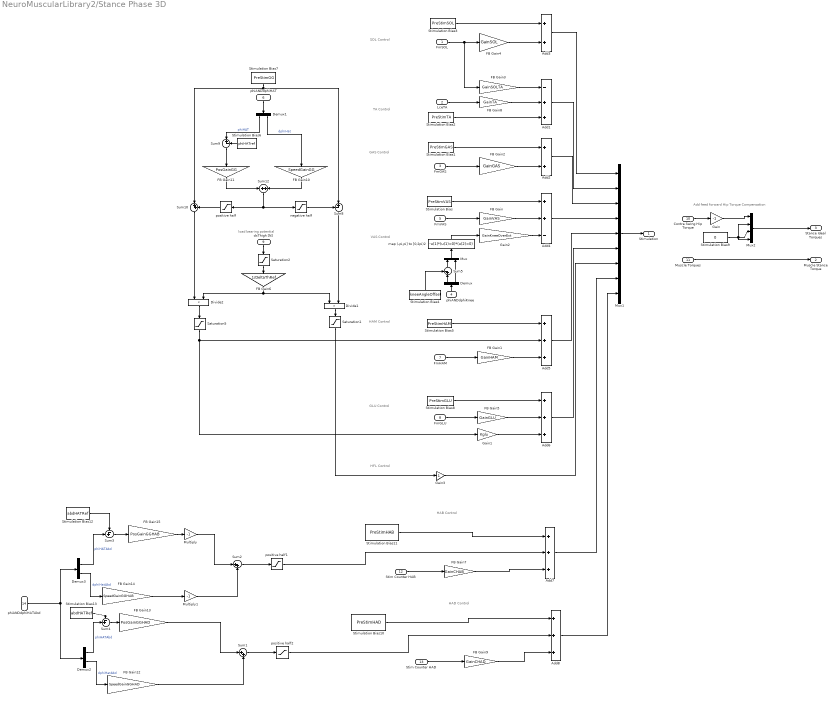
== system NeuroMuscularLibrary2/Stance Phase 3D ==
  note: Add feed forward Hip Torque Compensation
  note: load bearing potential
  note: HFL Control
  note: GLU Control
  note: VAS Control
  note: HAM Control
  note: GAS Control
  note: TA Control
  note: SOL Control
  note: HAB Control
  note: HAD Control
  FmSOL : Inport
  LceTA : Inport  Port=2
  FmGAS : Inport  Port=3
  phiANDdphiKnee : Inport  Port=4
  FmVAS : Inport  Port=5
  phiANDdphiHAT : Inport  Port=6
  FmHAM : Inport  Port=7
  FmGLU : Inport  Port=8
  dxThigh [N] : Inport  Port=9
  Contra Swing Hip Torque : Inport  Port=10
  Muscle Torques : Inport  Port=11
  Stim Counter HAB : Inport  Port=12
  Stim Counter HAD : Inport  Port=13
  phiANDdphiHATAbd : Inport  Port=14
  Add1 : Sum  Inputs=-++
  Add2 : Sum
  Add3 : Sum
  Add4 : Sum  Inputs=++-
  Add{5..8} (4 alike) : Sum  Inputs=+++
  Demux{,1..3} (4 alike) : Demux  Outputs=2
  Divide1 : Product
  Divide2 : Product
  FB Gain : Gain  Gain=GainVAS  SaturateOnIntegerOverflow=on  OutDataTypeStr=Inherit: Same as input  ParamDataTypeStr=Inherit: Same as input
  FB Gain1 : Gain  Gain=GainHAM  SaturateOnIntegerOverflow=on  OutDataTypeStr=Inherit: Same as input  ParamDataTypeStr=Inherit: Same as input
  FB Gain10 : Gain  Gain=SpeedGainGG  SaturateOnIntegerOverflow=on  OutDataTypeStr=Inherit: Same as input  ParamDataTypeStr=Inherit: Same as input
  FB Gain11 : Gain  Gain=PosGainGG  SaturateOnIntegerOverflow=on  OutDataTypeStr=Inherit: Same as input  ParamDataTypeStr=Inherit: Same as input
  FB Gain12 : Gain  Gain=SpeedGainGGHAD  SaturateOnIntegerOverflow=on  OutDataTypeStr=Inherit: Same as input  ParamDataTypeStr=Inherit: Same as input
  FB Gain13 : Gain  Gain=PosGainGGHAD  SaturateOnIntegerOverflow=on  OutDataTypeStr=Inherit: Same as input  ParamDataTypeStr=Inherit: Same as input
  FB Gain14 : Gain  Gain=SpeedGainGGHAB  SaturateOnIntegerOverflow=on  OutDataTypeStr=Inherit: Same as input  ParamDataTypeStr=Inherit: Same as input
  FB Gain15 : Gain  Gain=PosGainGGHAB  SaturateOnIntegerOverflow=on  OutDataTypeStr=Inherit: Same as input  ParamDataTypeStr=Inherit: Same as input
  FB Gain2 : Gain  Gain=GainGAS  SaturateOnIntegerOverflow=on  OutDataTypeStr=Inherit: Same as input  ParamDataTypeStr=Inherit: Same as input
  FB Gain3 : Gain  Gain=GainSOLTA  SaturateOnIntegerOverflow=on  OutDataTypeStr=Inherit: Same as input  ParamDataTypeStr=Inherit: Same as input
  FB Gain4 : Gain  Gain=GainSOL  SaturateOnIntegerOverflow=on  OutDataTypeStr=Inherit: Same as input  ParamDataTypeStr=Inherit: Same as input
  FB Gain5 : Gain  Gain=GainGLU  SaturateOnIntegerOverflow=on  OutDataTypeStr=Inherit: Same as input  ParamDataTypeStr=Inherit: Same as input
  FB Gain6 : Gain  Gain=1/DeltaThRef  SaturateOnIntegerOverflow=on  OutDataTypeStr=Inherit: Same as input  ParamDataTypeStr=Inherit: Same as input
  FB Gain7 : Gain  Gain=GainCHAB  SaturateOnIntegerOverflow=on  OutDataTypeStr=Inherit: Same as input  ParamDataTypeStr=Inherit: Same as input
  FB Gain8 : Gain  Gain=GainTA  SaturateOnIntegerOverflow=on  OutDataTypeStr=Inherit: Same as input  ParamDataTypeStr=Inherit: Same as input
  FB Gain9 : Gain  Gain=GainCHAD  SaturateOnIntegerOverflow=on  OutDataTypeStr=Inherit: Same as input  ParamDataTypeStr=Inherit: Same as input
  Gain : Gain  Gain=-1
  Gain1 : Gain  Gain=Kglu
  Gain2 : Gain  Gain=GainKneeOverExt
  Gain3 : Gain
  Multiply : Gain  Gain=-1
  Multiply1 : Gain  Gain=-1
  Mux : Mux  Inputs=2
  Mux1 : Mux  Inputs=9
  Mux2 : Mux
  Saturation1 : Saturate  UpperLimit=1  LowerLimit=0  ZeroCross=off
  Saturation2 : Saturate  UpperLimit=inf  LowerLimit=0  ZeroCross=off
  Saturation5 : Saturate  UpperLimit=1  LowerLimit=0  ZeroCross=off
  Stimulation Bias : Constant  Value=PreStimVAS
  Stimulation Bias1 : Constant  Value=PreStimGAS
  Stimulation Bias10 : Constant  Value=PreStimHAD
  Stimulation Bias11 : Constant  Value=PreStimHAB
  Stimulation Bias12 : Constant  Value=abdHATRef
  Stimulation Bias13 : Constant  Value=abdHATRef
  Stimulation Bias2 : Constant  Value=PreStimTA
  Stimulation Bias3 : Constant  Value=PreStimSOL
  Stimulation Bias4 : Constant  Value=kneeAngleOffset
  Stimulation Bias5 : Constant  Value=PreStimHAM
  Stimulation Bias6 : Constant  Value=phiHATref
  Stimulation Bias7 : Constant  Value=PreStimGG
  Stimulation Bias8 : Constant  Value=PreStimGLU
  Stimulation Bias9 : Constant  Value=0
  Sum1 : Sum  Inputs=|++  SaturateOnIntegerOverflow=on  InputSameDT=on  OutDataTypeStr=Inherit: Same as first input
  Sum10 : Sum  Inputs=|++  SaturateOnIntegerOverflow=on  InputSameDT=on  OutDataTypeStr=Inherit: Same as first input
  Sum12 : Sum  SaturateOnIntegerOverflow=on  InputSameDT=on  OutDataTypeStr=Inherit: Same as first input
  Sum2 : Sum  Inputs=|++  SaturateOnIntegerOverflow=on  InputSameDT=on  OutDataTypeStr=Inherit: Same as first input
  Sum{3..5,8} (4 alike) : Sum  Inputs=-+|  SaturateOnIntegerOverflow=on  InputSameDT=on  OutDataTypeStr=Inherit: Same as first input
  Sum9 : Sum  Inputs=|+-  SaturateOnIntegerOverflow=on  InputSameDT=on  OutDataTypeStr=Inherit: Same as first input
  map (-pi,pi] to [0,2pi)2 : Fcn  Expr=-u(1)*(u(1)<0)*(u(2)<0)
  negative half : Saturate  UpperLimit=0  LowerLimit=-inf  ZeroCross=off
  positive half : Saturate  UpperLimit=inf  LowerLimit=0  ZeroCross=off
  positive half1 : Saturate  UpperLimit=inf  LowerLimit=0  ZeroCross=off
  positive half2 : Saturate  UpperLimit=inf  LowerLimit=0  ZeroCross=off
  Stimulation : Outport
  Muscle Stance Torque : Outport  Port=2
  Stance Ideal Torques : Outport  Port=3
  wires:
  Gain/1 -> Mux2/1
  Contra Swing Hip Torque/1 -> Gain/1
  Add4/1 -> Mux1/4
  Mux1/1 -> Stimulation/1
  Gain1/1 -> Add6/3
  FB Gain5/1 -> Add6/2
  Stimulation Bias8/1 -> Add6/1
  Add6/1 -> Mux1/6
  Add5/1 -> Mux1/5
  FB Gain1/1 -> Add5/3
  Stimulation Bias5/1 -> Add5/1
  Stimulation Bias/1 -> Add4/1
  Stimulation Bias1/1 -> Add2/1
  Add2/1 -> Mux1/3
  Stimulation Bias2/1 -> Add1/3
  Stimulation Bias3/1 -> Add3/1
  FmGLU/1 -> FB Gain5/1
  FmHAM/1 -> FB Gain1/1
  map (-pi,pi] to [0,2pi)2/1 -> Gain2/1
  Sum8/1 -> Divide1/2
  Sum10/1 -> Divide2/1
  Sum9/1 -> FB Gain11/1
  FB Gain6/1 -> Divide2/2, Divide1/1
  Saturation5/1 -> Add5/2, Gain1/1
  Divide2/1 -> Saturation5/1
  Divide1/1 -> Saturation1/1
  Saturation1/1 -> Gain3/1
  dxThigh [N]/1 -> Saturation2/1
  Saturation2/1 -> FB Gain6/1
  Gain3/1 -> Mux1/7
  Gain2/1 -> Add4/3
  negative half/1 -> Sum8/1
  Sum12/1 -> negative half/1, positive half/1
  positive half/1 -> Sum10/2
  Demux1/2 -> FB Gain10/1  "dphiHat"
  Demux1/1 -> Sum9/1  "phiHAT"
  phiANDdphiHAT/1 -> Demux1/1
  FB Gain10/1 -> Sum12/2
  FB Gain11/1 -> Sum12/1
  Stimulation Bias7/1 -> Sum8/2, Sum10/1
  Stimulation Bias6/1 -> Sum9/2
  Stimulation Bias4/1 -> Sum5/1
  Demux/2 -> Mux/2
  Demux/1 -> Sum5/2
  phiANDdphiKnee/1 -> Demux/1
  Sum5/1 -> Mux/1
  Mux/1 -> map (-pi,pi] to [0,2pi)2/1
  FmVAS/1 -> FB Gain/1
  FB Gain/1 -> Add4/2
  FB Gain2/1 -> Add2/2
  FmGAS/1 -> FB Gain2/1
  LceTA/1 -> FB Gain8/1
  FB Gain8/1 -> Add1/2
  Add1/1 -> Mux1/2
  FB Gain3/1 -> Add1/1
  FmSOL/1 -> FB Gain3/1, FB Gain4/1
  FB Gain4/1 -> Add3/2
  Add3/1 -> Mux1/1
  Stimulation Bias9/1 -> Mux2/4, Mux2/3, Mux2/2
  Mux2/1 -> Stance Ideal Torques/1
  Muscle Torques/1 -> Muscle Stance Torque/1
  Stim Counter HAB/1 -> FB Gain7/1
  Stim Counter HAD/1 -> FB Gain9/1
  Demux3/1 -> Sum3/2  "phiHATAbd"
  Demux3/2 -> FB Gain14/1  "dphiHatAbd"
  Stimulation Bias11/1 -> Add7/1
  FB Gain7/1 -> Add7/3
  FB Gain9/1 -> Add8/3
  Add7/1 -> Mux1/8
  Add8/1 -> Mux1/9
  FB Gain15/1 -> Multiply/1
  FB Gain14/1 -> Multiply1/1
  Multiply1/1 -> Sum2/2
  Multiply/1 -> Sum2/1
  Sum2/1 -> positive half1/1
  positive half1/1 -> Add7/2
  Demux2/2 -> FB Gain12/1  "dphiHatAbd"
  FB Gain13/1 -> Sum1/1
  phiANDdphiHATAbd/1 -> Demux3/1, Demux2/1
  FB Gain12/1 -> Sum1/2
  Sum1/1 -> positive half2/1
  Demux2/1 -> Sum4/2  "phiHATAbd"
  positive half2/1 -> Add8/2
  Stimulation Bias10/1 -> Add8/1
  Sum3/1 -> FB Gain15/1
  Stimulation Bias12/1 -> Sum3/1
  Stimulation Bias13/1 -> Sum4/1
  Sum4/1 -> FB Gain13/1

== system NeuroMuscularLibrary2/Stimulation Mixing ==
  Stance Stim : Inport
  dxThigh : Inport  Port=2
  Stance? : Inport  Port=3
  ContraLegLeading? : Inport  Port=4
  Swing Stim : Inport  Port=5
  Constant : Constant
  FB Gain1 : Gain  Gain=1/DeltaThRef  SaturateOnIntegerOverflow=on  OutDataTypeStr=Inherit: Same as input  ParamDataTypeStr=Inherit: Same as input
  Logical Operator : Logic  Operator=NOT  AllPortsSameDT=off  OutDataTypeStr=boolean
  Logical Operator1 : Logic  Operator=NOT  AllPortsSameDT=off  OutDataTypeStr=boolean
  Product{,1..3} (4 alike) : Product
  Product4 : Product  Inputs=3
  Saturation17 : Saturate  UpperLimit=1  LowerLimit=0.01  ZeroCross=off
  Saturation2 : Saturate  UpperLimit=1  LowerLimit=0  ZeroCross=off
  Sum : Sum  Inputs=+|+
  Sum1 : Sum  Inputs=-+|
  Sum3 : Sum  Inputs=+++
  stimulation : Outport  OutputWhenDisabled=reset
  wires:
  dxThigh/1 -> FB Gain1/1
  Stance Stim/1 -> Product4/1, Product/1
  FB Gain1/1 -> Saturation2/1
  Saturation2/1 -> Product/2, Sum1/1
  Swing Stim/1 -> Product3/1, Product1/2
  Constant/1 -> Sum1/2
  Sum1/1 -> Product1/1
  Product1/1 -> Sum/2
  Product/1 -> Sum/1
  Logical Operator/1 -> Product4/3
  Stance?/1 -> Logical Operator1/1, Product4/2
  Sum/1 -> Product2/1
  Product2/1 -> Sum3/2  "Mixed Stimulation"
  Sum3/1 -> Saturation17/1
  Saturation17/1 -> stimulation/1
  Product4/1 -> Sum3/1  "Stance Stimulation Only"
  Logical Operator1/1 -> Product3/2
  Product3/1 -> Sum3/3  "Swing Stimulation Only"
  ContraLegLeading?/1 -> Product2/2, Logical Operator/1

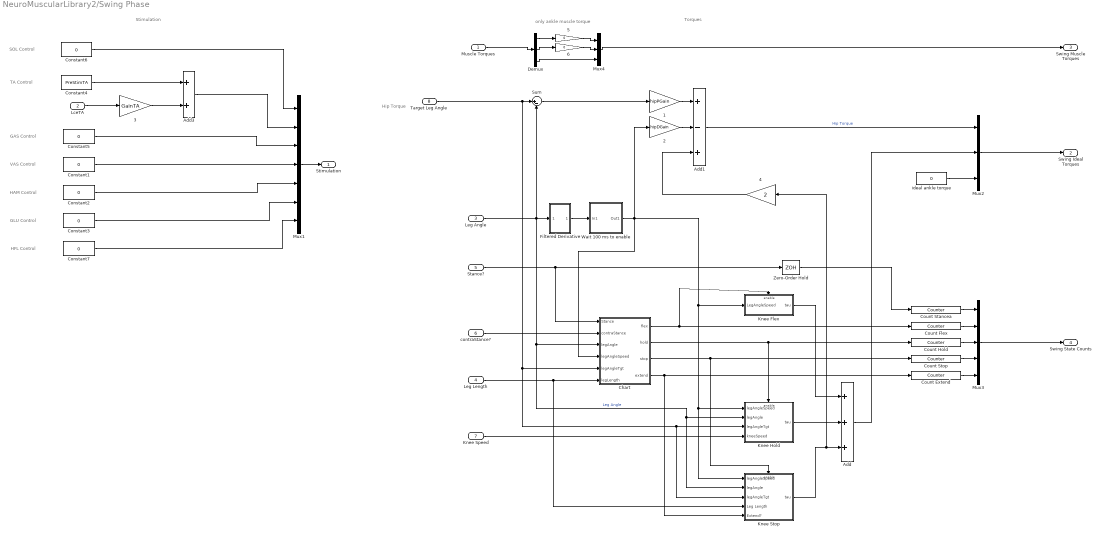
== system NeuroMuscularLibrary2/Swing Phase ==
  note: Stimulation
  note: SOL Control
  note: GAS Control
  note: TA Control
  note: VAS Control
  note: HAM Control
  note: GLU Control
  note: HFL Control
  note: Torques
  note: Hip Torque
  note: only ankle muscle torque
  Muscle Torques : Inport
  LceTA : Inport  Port=2
  Leg Angle : Inport  Port=3
  Leg Length : Inport  Port=4
  Stance? : Inport  Port=5
  contraStance? : Inport  Port=6
  Knee Speed : Inport  Port=7
  Target Leg Angle : Inport  Port=8
  " 1" : Gain  Gain=hipPGain
  " 2" : Gain  Gain=hipDGain
  " 3" : Gain  Gain=GainTA
  " 4" : Gain  Gain=2
  " 5" : Gain  Gain=0
  " 6" : Gain  Gain=0
  Add : Sum  Inputs=+++
  Add1 : Sum  Inputs=+-+
  Add3 : Sum
  Chart : Stateflow chart  TreatAsAtomicUnit=on
  Constant{1..3,5..7} (6 alike) : Constant  Value=0
  Constant4 : Constant  Value=PreStimTA
  Count Extend : dspswit3/Counter  Direction=Up  CountEvent=Rising edge  CounterSize=16 bits  MaxCount=255  InitialCount=0  Output=Count  HitValue=32  ResetInput=off  SamplesPerFrame=1  Ts=1  CntDtype=double  HitDtype=Logical
  Count Flex : dspswit3/Counter  Direction=Up  CountEvent=Rising edge  CounterSize=16 bits  MaxCount=255  InitialCount=0  Output=Count  HitValue=32  ResetInput=off  SamplesPerFrame=1  Ts=1  CntDtype=double  HitDtype=Logical
  Count Hold : dspswit3/Counter  Direction=Up  CountEvent=Rising edge  CounterSize=16 bits  MaxCount=255  InitialCount=0  Output=Count  HitValue=32  ResetInput=off  SamplesPerFrame=1  Ts=1  CntDtype=double  HitDtype=Logical
  Count Stancea : dspswit3/Counter  Direction=Up  CountEvent=Rising edge  CounterSize=16 bits  MaxCount=255  InitialCount=0  Output=Count  HitValue=32  ResetInput=off  SamplesPerFrame=1  Ts=1  CntDtype=double  HitDtype=Logical
  Count Stop : dspswit3/Counter  Direction=Up  CountEvent=Rising edge  CounterSize=16 bits  MaxCount=255  InitialCount=0  Output=Count  HitValue=32  ResetInput=off  SamplesPerFrame=1  Ts=1  CntDtype=double  HitDtype=Logical
  Demux : Demux  Outputs=3
  Filtered Derivative : Subsystem
  Knee Flex : Subsystem  TreatAsAtomicUnit=on
  Knee Hold : Subsystem  TreatAsAtomicUnit=on
  Knee Stop : Subsystem  TreatAsAtomicUnit=on
  Mux1 : Mux  Inputs=7
  Mux2 : Mux  Inputs=3
  Mux3 : Mux  Inputs=5
  Mux4 : Mux  Inputs=3
  Sum : Sum  Inputs=|+-
  Wait 100 ms to enable : Subsystem
  Zero-Order Hold : ZeroOrderHold  SampleTime=.01
  ideal ankle torque : Constant  Value=0
  Stimulation : Outport
  Swing Ideal Torques : Outport  Port=2
  Swing Muscle Torques : Outport  Port=3
  Swing State Counts : Outport  Port=4
  wires:
  Demux/3 -> Mux4/3
  " 6"/1 -> Mux4/2
  " 5"/1 -> Mux4/1
  Demux/2 -> " 6"/1
  Demux/1 -> " 5"/1
  Muscle Torques/1 -> Demux/1
  Mux4/1 -> Swing Muscle Torques/1
  Mux2/1 -> Swing Ideal Torques/1
  ideal ankle torque/1 -> Mux2/3
  Zero-Order Hold/1 -> Count Stancea/1
  Count Stancea/1 -> Mux3/1
  Mux3/1 -> Swing State Counts/1
  Count Flex/1 -> Mux3/2
  Count Hold/1 -> Mux3/3
  Count Stop/1 -> Mux3/4
  Count Extend/1 -> Mux3/5
  Add1/1 -> Mux2/1  "Hip Torque"
  Leg Length/1 -> Knee Stop/4(Leg Length), Chart/6(legLength)
  contraStance?/1 -> Chart/2(contraStance)
  Stance?/1 -> Chart/1(Stance), Zero-Order Hold/1
  Chart/4(extend) -> Knee Stop/5(Extend?), Count Extend/1
  Chart/3(stop) -> Knee Stop/Enable, Count Stop/1
  Chart/2(hold) -> Knee Hold/Enable, Count Hold/1
  Chart/1(flex) -> Count Flex/1, Knee Flex/Enable
  " 4"/1 -> Add1/3
  Add/1 -> Mux2/2
  Knee Stop/1(tau) -> Add/3, " 4"/1
  Knee Flex/1(tau) -> Add/1
  Knee Hold/1(tau) -> Add/2
  Knee Speed/1 -> Knee Hold/4(kneeSpeed)
  Constant4/1 -> Add3/1
  " 3"/1 -> Add3/2
  LceTA/1 -> " 3"/1
  Add3/1 -> Mux1/2
  Constant6/1 -> Mux1/1
  Constant5/1 -> Mux1/3
  Constant1/1 -> Mux1/4
  Constant2/1 -> Mux1/5
  Constant3/1 -> Mux1/6
  Constant7/1 -> Mux1/7
  Mux1/1 -> Stimulation/1
  Leg Angle/1 -> Sum/2, Knee Hold/2(legAngle), Knee Stop/2(legAngle), Chart/3(legAngle), Filtered Derivative/1(In1)  "Leg Angle"
  Sum/1 -> " 1"/1
  " 1"/1 -> Add1/1
  " 2"/1 -> Add1/2
  Target Leg Angle/1 -> Knee Hold/3(legAngleTgt), Knee Stop/3(legAngleTgt), Chart/5(legAngleTgt), Sum/1
  Filtered Derivative/1(Out1) -> Wait 100 ms to enable/1(In1)
  Wait 100 ms to enable/1(Out1) -> " 2"/1, Knee Flex/1(LegAngleSpeed), Knee Stop/1(legAngleSpeed), Knee Hold/1(legAngleSpeed), Chart/4(legAngleSpeed)
